simulink model "svpwm_2"  (R2020a)
settings: Solver=VariableStepAuto  StartTime=0.0  StopTime=1  RelTol=1e-3
libraries: simulink x12, powerlib x1
settings Model: Creator=hp  LastModifiedBy=hp

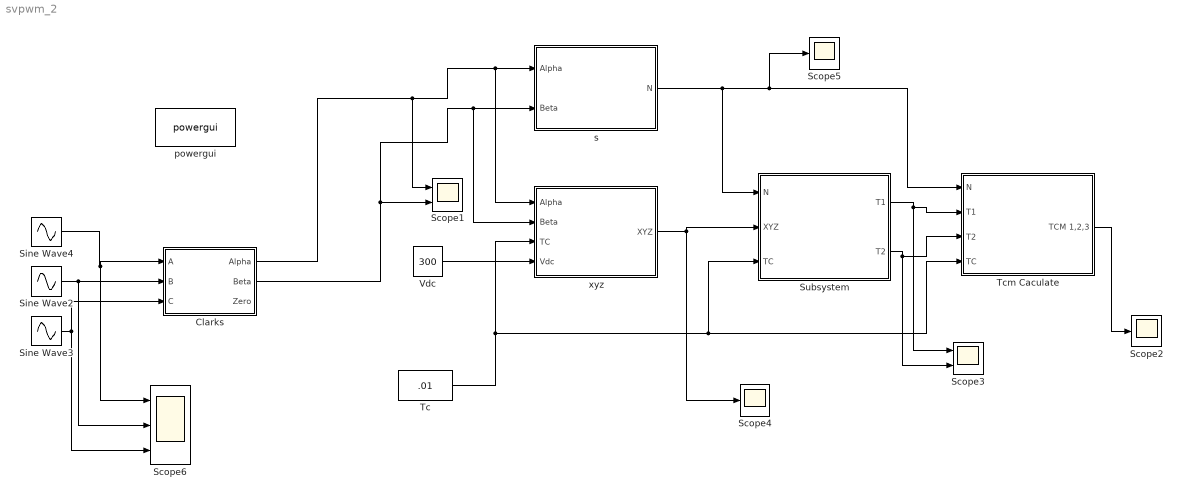
== system svpwm_2 ==
  Clarks : Subsystem
  Scope1 : Scope  NumInputPorts=2
  Scope2 : Scope
  Scope3 : Scope  NumInputPorts=2
  Scope4 : Scope
  Scope5 : Scope
  Scope6 : Scope  NumInputPorts=3
  Sine Wave2 : Sin  Amplitude=30  Frequency=2*pi*50  Phase=(2*pi)/3  SampleTime=5e-6
  Sine Wave3 : Sin  Amplitude=30  Frequency=2*pi*50  Phase=(4*pi)/3  SampleTime=5e-6
  Sine Wave4 : Sin  Amplitude=30  Frequency=2*pi*50  SampleTime=5e-6
  Subsystem : Subsystem
  Tc : Constant  Value=.01
  Tcm Caculate : Subsystem
  Vdc : Constant  Value=300
  powergui : powerlib/powergui  Priority=1  SimulationMode=Discrete  SampleTime=50e-6  frequency=60  Iterations=50  frequencyindice=60  Pbase=100e6  ErrMax=1e-4  UnitsV=kV  UnitsW=MW  buscounter=0  FunctionMessages=off  echomessages=off  EnableUseOfTLC=off  CurrentSourceSwitches=off  DisableSnubberDevices=off  DisableRonSwitches=off  DisableVfSwitches=off  DisplayEquations=off  AutomaticDiscreteSolvers=off  SolverType=Tustin/Backward Euler (TBE)  Interpol=off  ExternalGateDelay=off  methode=off  Ts=100  x0status=blocks  SPID=on  SwTol=0  HookPort=off  NonlinearTolerance=1e-4  nMaxIteration=100  ContinueOnMaxIteration=off  RestoreLinks=warning  ResistiveCurrentMeasurement=off  Frange=[0:2:500]  Ylog=off  Xlog=on  ShowGrid=off  save=off  variable=ZData  structure=0  ZoomFFT=off  StartTime=0.0  cycles=1  DisplayStyle=1  fundamental=60  FreqAxis=off  MaxFrequency=1000  frequencyindicesteady=1  RmsSteady=1  display=off
  s : Subsystem
  xyz : Subsystem
  wires:
  Tcm Caculate/1(TCM 1,2,3) -> Scope2/1
  Subsystem/1(T1) -> Scope3/1, Tcm Caculate/2(T1)
  Subsystem/2(T2) -> Scope3/2, Tcm Caculate/3(T2)
  Clarks/1(Alpha) -> Scope1/1, xyz/1(Alpha), s/1(Alpha)
  Tc/1 -> Tcm Caculate/4(TC), Subsystem/3(TC), xyz/3(TC)
  s/1(N) -> Subsystem/1(N), Scope5/1, Tcm Caculate/1(N)
  xyz/1(XYZ) -> Scope4/1, Subsystem/2(XYZ)
  Vdc/1 -> xyz/4(Vdc)
  Clarks/2(Beta) -> xyz/2(Beta), s/2(Beta), Scope1/2
  Sine Wave2/1 -> Scope6/2, Clarks/2(B)
  Sine Wave3/1 -> Scope6/3, Clarks/3(C)
  Sine Wave4/1 -> Scope6/1, Clarks/1(A)

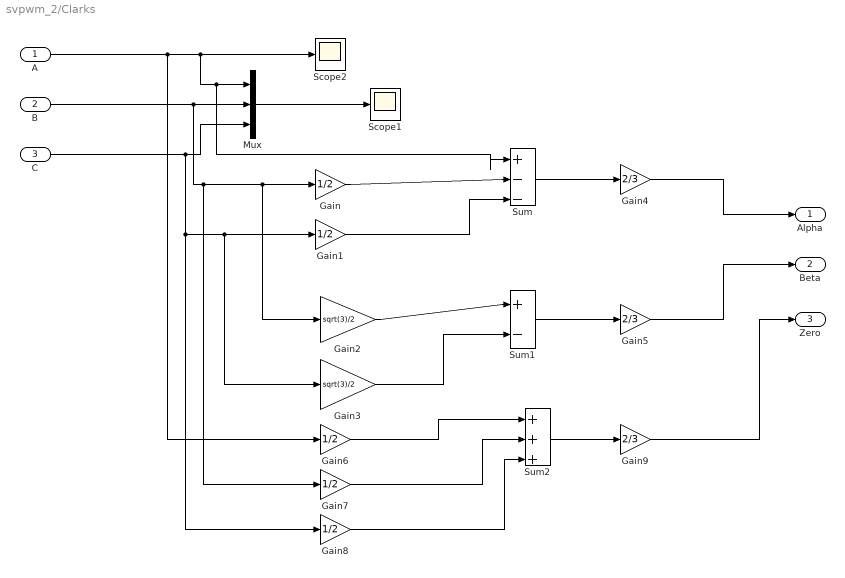
== system svpwm_2/Clarks ==
  A : Inport
  B : Inport  Port=2
  C : Inport  Port=3
  Gain{,1,6..8} (5 alike) : Gain  Gain=1/2
  Gain2 : Gain  Gain=sqrt(3)/2
  Gain3 : Gain  Gain=sqrt(3)/2
  Gain4 : Gain  Gain=2/3
  Gain5 : Gain  Gain=2/3
  Gain9 : Gain  Gain=2/3
  Mux : Mux  Inputs=3
  Scope1 : Scope
  Scope2 : Scope
  Sum : Sum  Inputs=|+--
  Sum1 : Sum  Inputs=|+-
  Sum2 : Sum  Inputs=|+++
  Alpha : Outport
  Beta : Outport  Port=2
  Zero : Outport  Port=3
  wires:
  A/1 -> Gain6/1, Sum/1, Mux/1, Scope2/1
  Gain8/1 -> Sum2/3
  Mux/1 -> Scope1/1
  Gain/1 -> Sum/2
  Gain4/1 -> Alpha/1
  Gain3/1 -> Sum1/2
  B/1 -> Gain7/1, Gain2/1, Gain/1, Mux/2
  C/1 -> Gain8/1, Gain3/1, Gain1/1, Mux/3
  Sum1/1 -> Gain5/1
  Gain7/1 -> Sum2/2
  Gain2/1 -> Sum1/1
  Sum2/1 -> Gain9/1
  Gain6/1 -> Sum2/1
  Sum/1 -> Gain4/1
  Gain1/1 -> Sum/3
  Gain5/1 -> Beta/1
  Gain9/1 -> Zero/1

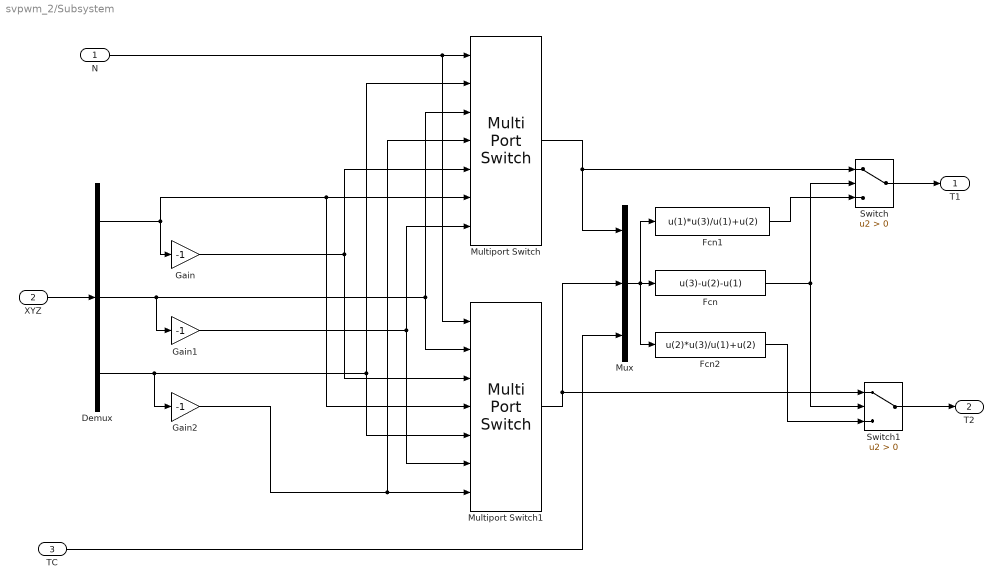
== system svpwm_2/Subsystem ==
  N : Inport
  XYZ : Inport  Port=2
  TC : Inport  Port=3
  Demux : Demux  Outputs=3
  Fcn : Fcn  Expr=u(3)-u(2)-u(1)
  Fcn1 : Fcn  Expr=u(1)*u(3)/u(1)+u(2)
  Fcn2 : Fcn  Expr=u(2)*u(3)/u(1)+u(2)
  Gain : Gain  Gain=-1
  Gain1 : Gain  Gain=-1
  Gain2 : Gain  Gain=-1
  Multiport Switch : MultiPortSwitch  Inputs=6
  Multiport Switch1 : MultiPortSwitch  Inputs=6
  Mux : Mux  Inputs=3
  Switch : Switch  Criteria=u2 > Threshold
  Switch1 : Switch  Criteria=u2 > Threshold
  T1 : Outport
  T2 : Outport  Port=2
  wires:
  XYZ/1 -> Demux/1
  N/1 -> Multiport Switch1/1, Multiport Switch/1
  Demux/2 -> Gain1/1, Multiport Switch1/2, Multiport Switch/3
  Gain1/1 -> Multiport Switch1/6, Multiport Switch/7
  Demux/3 -> Gain2/1, Multiport Switch/2, Multiport Switch1/5
  Gain2/1 -> Multiport Switch1/7, Multiport Switch/4
  Demux/1 -> Gain/1, Multiport Switch1/4, Multiport Switch/6
  Gain/1 -> Multiport Switch1/3, Multiport Switch/5
  TC/1 -> Mux/3
  Multiport Switch1/1 -> Switch1/1, Mux/2
  Multiport Switch/1 -> Switch/1, Mux/1
  Mux/1 -> Fcn1/1, Fcn2/1, Fcn/1
  Fcn/1 -> Switch1/2, Switch/2
  Switch1/1 -> T2/1
  Switch/1 -> T1/1
  Fcn1/1 -> Switch/3
  Fcn2/1 -> Switch1/3

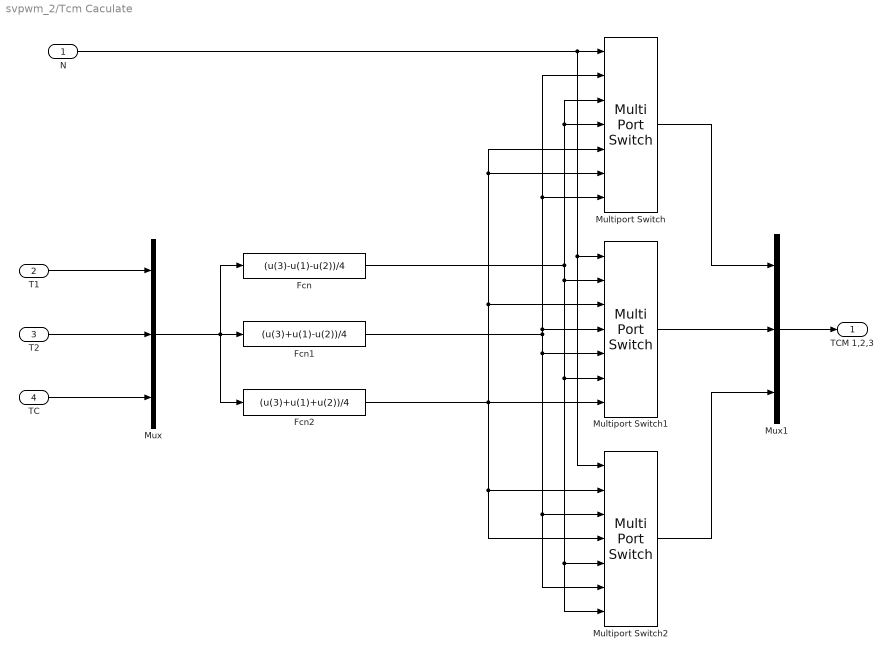
== system svpwm_2/Tcm Caculate ==
  N : Inport
  T1 : Inport  Port=2
  T2 : Inport  Port=3
  TC : Inport  Port=4
  Fcn : Fcn  Expr=(u(3)-u(1)-u(2))/4
  Fcn1 : Fcn  Expr=(u(3)+u(1)-u(2))/4
  Fcn2 : Fcn  Expr=(u(3)+u(1)+u(2))/4
  Multiport Switch : MultiPortSwitch  Inputs=6
  Multiport Switch1 : MultiPortSwitch  Inputs=6
  Multiport Switch2 : MultiPortSwitch  Inputs=6
  Mux : Mux  Inputs=3
  Mux1 : Mux  Inputs=3
  TCM 1,2,3 : Outport
  wires:
  T1/1 -> Mux/1
  T2/1 -> Mux/2
  TC/1 -> Mux/3
  Mux/1 -> Fcn2/1, Fcn1/1, Fcn/1
  Multiport Switch1/1 -> Mux1/2
  Multiport Switch2/1 -> Mux1/3
  Multiport Switch/1 -> Mux1/1
  Mux1/1 -> TCM 1,2,3/1
  N/1 -> Multiport Switch2/1, Multiport Switch1/1, Multiport Switch/1
  Fcn/1 -> Multiport Switch2/7, Multiport Switch2/5, Multiport Switch1/6, Multiport Switch1/2, Multiport Switch/4, Multiport Switch/3
  Fcn1/1 -> Multiport Switch2/6, Multiport Switch2/3, Multiport Switch1/5, Multiport Switch1/4, Multiport Switch/2, Multiport Switch/7
  Fcn2/1 -> Multiport Switch/5, Multiport Switch/6, Multiport Switch1/3, Multiport Switch1/7, Multiport Switch2/4, Multiport Switch2/2

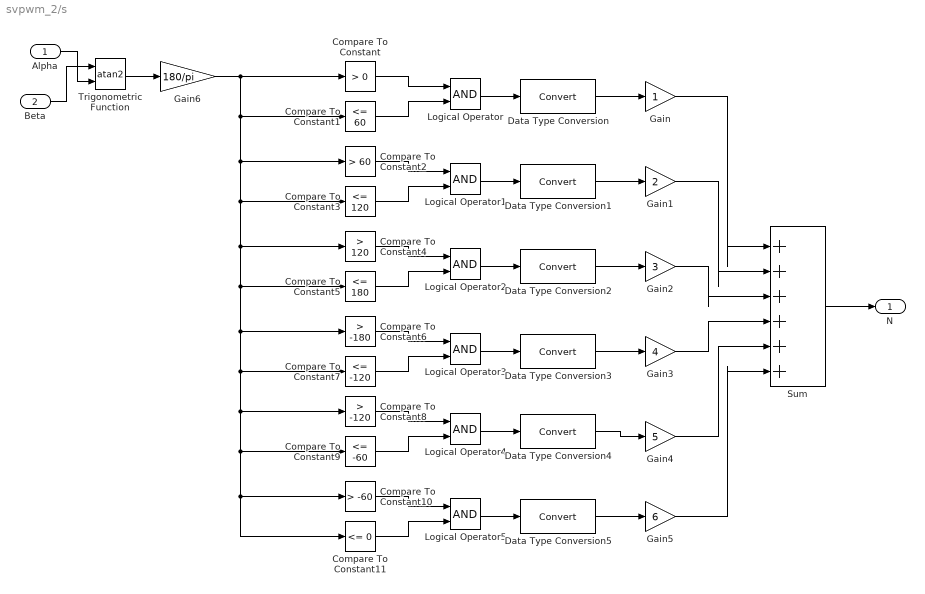
== system svpwm_2/s ==
  Alpha : Inport
  Beta : Inport  Port=2
  Compare To Constant : simulink/Logic and Bit Operations/Compare To Constant  relop=>  const=0  OutDataTypeStr=boolean
  Compare To Constant1 : simulink/Logic and Bit Operations/Compare To Constant  relop=<=  const=60  OutDataTypeStr=boolean
  Compare To Constant10 : simulink/Logic and Bit Operations/Compare To Constant  relop=>  const=-60  OutDataTypeStr=boolean
  Compare To Constant11 : simulink/Logic and Bit Operations/Compare To Constant  relop=<=  const=0  OutDataTypeStr=boolean
  Compare To Constant2 : simulink/Logic and Bit Operations/Compare To Constant  relop=>  const=60  OutDataTypeStr=boolean
  Compare To Constant3 : simulink/Logic and Bit Operations/Compare To Constant  relop=<=  const=120  OutDataTypeStr=boolean
  Compare To Constant4 : simulink/Logic and Bit Operations/Compare To Constant  relop=>  const=120  OutDataTypeStr=boolean
  Compare To Constant5 : simulink/Logic and Bit Operations/Compare To Constant  relop=<=  const=180  OutDataTypeStr=boolean
  Compare To Constant6 : simulink/Logic and Bit Operations/Compare To Constant  relop=>  const=-180  OutDataTypeStr=boolean
  Compare To Constant7 : simulink/Logic and Bit Operations/Compare To Constant  relop=<=  const=-120  OutDataTypeStr=boolean
  Compare To Constant8 : simulink/Logic and Bit Operations/Compare To Constant  relop=>  const=-120  OutDataTypeStr=boolean
  Compare To Constant9 : simulink/Logic and Bit Operations/Compare To Constant  relop=<=  const=-60  OutDataTypeStr=boolean
  Data Type Conversion{,1..5} (6 alike) : DataTypeConversion
  Gain : Gain
  Gain1 : Gain  Gain=2
  Gain2 : Gain  Gain=3
  Gain3 : Gain  Gain=4
  Gain4 : Gain  Gain=5
  Gain5 : Gain  Gain=6
  Gain6 : Gain  Gain=180/pi
  Logical Operator{,1..5} (6 alike) : Logic  AllPortsSameDT=off  OutDataTypeStr=boolean
  Sum : Sum  Inputs=|++++++
  Trigonometric Function : Trigonometry  Operator=atan2
  N : Outport
  wires:
  Beta/1 -> Trigonometric Function/1
  Alpha/1 -> Trigonometric Function/2
  Compare To Constant/1 -> Logical Operator/1
  Compare To Constant1/1 -> Logical Operator/2
  Logical Operator/1 -> Data Type Conversion/1
  Logical Operator1/1 -> Data Type Conversion1/1
  Compare To Constant3/1 -> Logical Operator1/2
  Compare To Constant2/1 -> Logical Operator1/1
  Compare To Constant4/1 -> Logical Operator2/1
  Compare To Constant5/1 -> Logical Operator2/2
  Logical Operator2/1 -> Data Type Conversion2/1
  Logical Operator3/1 -> Data Type Conversion3/1
  Compare To Constant7/1 -> Logical Operator3/2
  Compare To Constant6/1 -> Logical Operator3/1
  Compare To Constant8/1 -> Logical Operator4/1
  Compare To Constant9/1 -> Logical Operator4/2
  Logical Operator4/1 -> Data Type Conversion4/1
  Logical Operator5/1 -> Data Type Conversion5/1
  Compare To Constant11/1 -> Logical Operator5/2
  Compare To Constant10/1 -> Logical Operator5/1
  Trigonometric Function/1 -> Gain6/1
  Data Type Conversion/1 -> Gain/1
  Data Type Conversion1/1 -> Gain1/1
  Data Type Conversion2/1 -> Gain2/1
  Data Type Conversion3/1 -> Gain3/1
  Data Type Conversion4/1 -> Gain4/1
  Data Type Conversion5/1 -> Gain5/1
  Gain/1 -> Sum/1
  Gain1/1 -> Sum/2
  Gain2/1 -> Sum/3
  Gain3/1 -> Sum/4
  Gain4/1 -> Sum/5
  Gain5/1 -> Sum/6
  Sum/1 -> N/1
  Gain6/1 -> Compare To Constant5/1, Compare To Constant6/1, Compare To Constant10/1, Compare To Constant11/1, Compare To Constant9/1, Compare To Constant8/1, Compare To Constant7/1, Compare To Constant4/1, Compare To Constant3/1, Compare To Constant2/1, Compare To Constant1/1, Compare To Constant/1

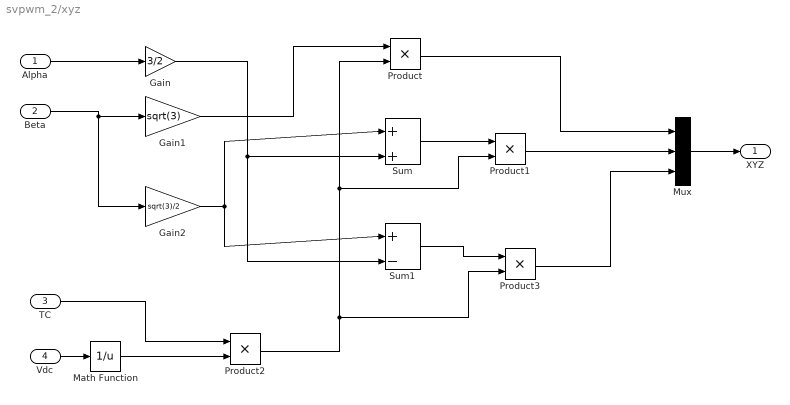
== system svpwm_2/xyz ==
  Alpha : Inport
  Beta : Inport  Port=2
  TC : Inport  Port=3
  Vdc : Inport  Port=4
  Gain : Gain  Gain=3/2
  Gain1 : Gain  Gain=sqrt(3)
  Gain2 : Gain  Gain=sqrt(3)/2
  Math Function : Math  Operator=reciprocal  SignedPower=on  RndMeth=Zero  SaturateOnIntegerOverflow=on
  Mux : Mux  Inputs=3
  Product{,1..3} (4 alike) : Product
  Sum : Sum  Inputs=|++
  Sum1 : Sum  Inputs=|+-
  XYZ : Outport
  wires:
  Vdc/1 -> Math Function/1
  TC/1 -> Product2/1
  Math Function/1 -> Product2/2
  Beta/1 -> Gain2/1, Gain1/1
  Alpha/1 -> Gain/1
  Gain1/1 -> Product/1
  Product2/1 -> Product3/2, Product1/2, Product/2
  Gain/1 -> Sum1/2, Sum/2
  Gain2/1 -> Sum/1, Sum1/1
  Sum/1 -> Product1/1
  Sum1/1 -> Product3/1
  Product/1 -> Mux/1
  Product1/1 -> Mux/2
  Product3/1 -> Mux/3
  Mux/1 -> XYZ/1
